simulink model "FSAE_ClosedLoop"  (R2026b)
settings: Solver=ode45  StopTime=Simulation.StopTimeSmoke.Value
undefined symbols (not defined in the file): DefaultEnvironmentBus, DefaultTrackReferenceBus
settings Model: DataDictionary=VehicleData.sldd  Creator=Xu Dingyi  LastModifiedBy=29358

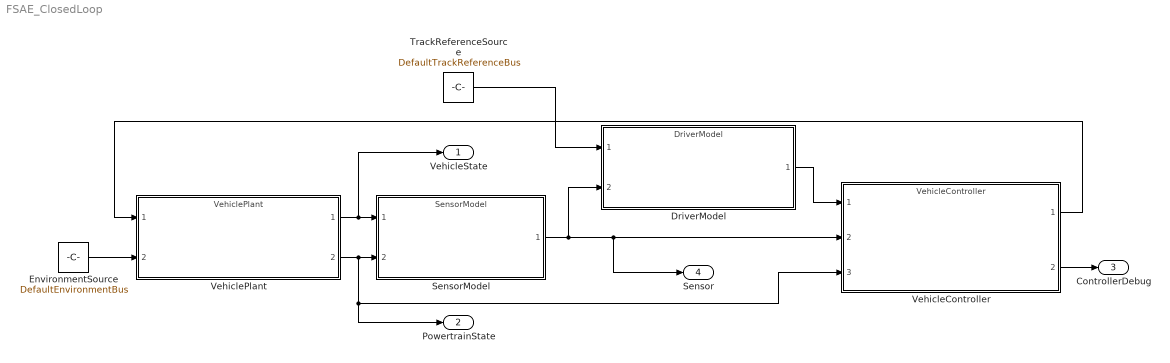
== system FSAE_ClosedLoop ==
  DriverModel : ModelReference  ModelNameDialog=DriverModel  SimulationMode=Normal  ModelReferenceVersion=2.0
  EnvironmentSource : Constant  Value=DefaultEnvironmentBus  OutDataTypeStr=Bus: EnvironmentBus  SampleTime=-1
  SensorModel : ModelReference  ModelNameDialog=SensorModel  SimulationMode=Normal  ModelReferenceVersion=2.0
  TrackReferenceSource : Constant  Value=DefaultTrackReferenceBus  OutDataTypeStr=Bus: TrackReferenceBus  SampleTime=-1
  VehicleController : ModelReference  ModelNameDialog=VehicleController  SimulationMode=Normal  ModelReferenceVersion=2.0
  VehiclePlant : ModelReference  ModelNameDialog=VehiclePlant  SimulationMode=Normal  ModelReferenceVersion=2.0
  VehicleState : Outport  OutDataTypeStr=Bus: VehicleStateBus
  PowertrainState : Outport  Port=2  OutDataTypeStr=Bus: PowertrainStateBus
  ControllerDebug : Outport  Port=3  OutDataTypeStr=Bus: ControllerDebugBus
  Sensor : Outport  Port=4  OutDataTypeStr=Bus: SensorBus
  wires:
  VehicleController/2 -> ControllerDebug/1
  VehiclePlant/1 -> SensorModel/1, VehicleState/1
  EnvironmentSource/1 -> VehiclePlant/2
  VehicleController/1 -> VehiclePlant/1
  VehiclePlant/2 -> VehicleController/3, PowertrainState/1, SensorModel/2
  DriverModel/1 -> VehicleController/1
  SensorModel/1 -> VehicleController/2, Sensor/1, DriverModel/2
  TrackReferenceSource/1 -> DriverModel/1
